simulink library "SimscapeCustomComponents_lib"  (R2025b)
settings: Solver=VariableStepAuto  StartTime=0.0  StopTime=10.0  RelTol=1e-3
undefined symbols (not defined in the file or in its folder): base, baseVdc, capacity, DiscIntNeverNeededParam, ee_sli_rtmsupport, filterInductance, freqeuncy, frequency, gcbh, gflInverter, gfmInverter, iMaxPU, Inertia, initialSOC, plantRating, solar, Ts, ups, Vac, windSystem, windTurbine
libraries: fl_lib x397, nesl_utility x171, eeGeneralControl x85, ee_lib x82, simulink x72, datacenter_lib x68, eeTransforms x38, slpidlib x24, buildingEnergy_lib x20, SimscapeFluids_lib x17, eeSinusoidalMeasurementV2 x8, eePwmGenerator x8
(part 23 of 24)

== system SimscapeCustomComponents_lib/Microgrid and Renewables/Sources/Solar Plant Integrated/Detailed/PV Plant & Controller/Controller/MPPT/Solar PV Controller/DC voltage controller & current reference/Current limits ==
  Imax : Inport
  idref : Inport  Port=2
  Sqrt1 : Sqrt
  Square3 : Math  Operator=square
  Square4 : Math  Operator=square
  Sum9 : Sum  Inputs=|+-
  iubd : Outport
  iubq : Outport  Port=2
  wires:
  Sum9/1 -> Sqrt1/1
  Square3/1 -> Sum9/1
  Square4/1 -> Sum9/2
  Imax/1 -> iubd/1, Square3/1
  Sqrt1/1 -> iubq/1
  idref/1 -> Square4/1

== system SimscapeCustomComponents_lib/Microgrid and Renewables/Sources/Solar Plant Integrated/Detailed/PV Plant & Controller/Controller/MPPT/Solar PV Controller/DC voltage controller & current reference/If Action Subsystem ==
  note: iq_ref_generator
  note: id_ref_generator
  Q ref : Inport
  Vmag : Inport  Port=2
  P pv : Inport  Port=3
  vdc : Inport  Port=4
  vdc ref : Inport  Port=5
  Action Port : ActionPort
  Subsystem : Subsystem
  Subsystem1 : Subsystem
  iq ref : Outport
  id ref : Outport  Port=2
  wires:
  [ubid] -> Subsystem1/5(id ub)
  [ubiq] -> Subsystem/2(iq ub)
  P pv/1 -> Subsystem1/2(P pv)
  Q ref/1 -> Subsystem/3(Q ref)
  vdc/1 -> Subsystem1/3(vdc)
  Vmag/1 -> Subsystem1/1(Vmag), Subsystem/1(V mag)
  vdc ref/1 -> Subsystem1/4(vdc ref)
  Subsystem1/1(idref) -> id ref/1
  Subsystem/1(iqref) -> iq ref/1

== system SimscapeCustomComponents_lib/Microgrid and Renewables/Sources/Solar Plant Integrated/Detailed/PV Plant & Controller/Controller/MPPT/Solar PV Controller/DC voltage controller & current reference/Subsystem ==
  V mag : Inport
  iq ub : Inport  Port=2
  Q ref : Inport  Port=3
  Constant : Constant  Value=1e-3
  Data Type Conversion Inherited : simulink/Signal Attributes/Data Type Conversion Inherited  ConvertRealWorld=Real World Value  DoSatur=off
  Divide2 : Product  Inputs=*/
  Gain1 : Gain  Gain=-1
  Gain3 : Gain  Gain=-1
  Saturation Dynamic2 : simulink/Discontinuities/Saturation Dynamic  OutMin=[]  OutMax=[]  OutDataTypeStr=Inherit: Same as second input  OutDataType=fixdt(1, 16)  OutScaling=2^-10  DoSatur=off
  Scope : Scope  NumInputPorts=3
      settings: ActiveDisplayYMinimum=1.32868  ActiveDisplayYMaximum=1.39248  DataLoggingVariableName=ScopeData8
  Switch : Switch  Criteria=u2 ~= 0  SaturateOnIntegerOverflow=off  InputSameDT=off
  iq ub1 : InportShadow  Port=2
  iqref : Outport
  wires:
  iq ub1/1 -> Gain3/1
  Divide2/1 -> Saturation Dynamic2/2, Scope/2
  Q ref/1 -> Divide2/1
  Gain3/1 -> Saturation Dynamic2/3, Scope/3
  iq ub/1 -> Saturation Dynamic2/1, Scope/1
  Saturation Dynamic2/1 -> Gain1/1
  V mag/1 -> Data Type Conversion Inherited/1, Switch/2, Switch/1
  Switch/1 -> Divide2/2
  Constant/1 -> Data Type Conversion Inherited/2
  Data Type Conversion Inherited/1 -> Switch/3
  Gain1/1 -> iqref/1

== system SimscapeCustomComponents_lib/Microgrid and Renewables/Sources/Solar Plant Integrated/Detailed/PV Plant & Controller/Controller/MPPT/Solar PV Controller/DC voltage controller & current reference/Subsystem1 ==
  Vmag : Inport
  P pv : Inport  Port=2
  vdc : Inport  Port=3
  vdc ref : Inport  Port=4
  id ub : Inport  Port=5
  Constant : Constant  Value=1e-3
  Constant4 : Constant  Value=0
  Data Type Conversion Inherited : simulink/Signal Attributes/Data Type Conversion Inherited  ConvertRealWorld=Real World Value  DoSatur=off
  Divide : Product  Inputs=/*
  Gain4 : Gain  Gain=1/(mVAbase)
  Saturation Dynamic1 : simulink/Discontinuities/Saturation Dynamic  OutMin=[]  OutMax=[]  OutDataTypeStr=Inherit: Same as second input  OutDataType=fixdt(1, 16)  OutScaling=2^-10  DoSatur=off
  Scope : Scope  NumInputPorts=2
      settings: ActiveDisplayYMinimum=715.83213  ActiveDisplayYMaximum=1444.49375
  Scope1 : Scope  NumInputPorts=3
      settings: ActiveDisplayYMinimum=0.2  ActiveDisplayYMaximum=2.2  DataLoggingVariableName=ScopeData7
  Sum : Sum  Inputs=|++
  Switch : Switch  Criteria=u2 ~= 0  SaturateOnIntegerOverflow=off  InputSameDT=off
  V_dc_Controller1 : Subsystem
  idref : Outport
  wires:
  Constant4/1 -> Saturation Dynamic1/3
  P pv/1 -> Gain4/1
  V_dc_Controller1/1(Out1) -> Sum/2
  Sum/1 -> Saturation Dynamic1/2, Scope1/2
  vdc ref/1 -> V_dc_Controller1/2(vdc ref), Scope/2
  id ub/1 -> Scope1/1, Saturation Dynamic1/1
  Gain4/1 -> Divide/2
  Divide/1 -> Sum/1
  Saturation Dynamic1/1 -> idref/1, Scope1/3
  vdc/1 -> V_dc_Controller1/1(vdc), Scope/1
  Vmag/1 -> Data Type Conversion Inherited/1, Switch/2, Switch/1
  Switch/1 -> Divide/1
  Constant/1 -> Data Type Conversion Inherited/2
  Data Type Conversion Inherited/1 -> Switch/3

== system SimscapeCustomComponents_lib/Microgrid and Renewables/Sources/Solar Plant Integrated/Detailed/PV Plant & Controller/Controller/MPPT/Solar PV Controller/PLL & Measurements/Subsystem ==
  abc : Inport
  Demux : Demux  Outputs=3
  Park Transform : eeTransforms/Park Transform  AxisAlignment=Q-axis  PowerInvariant=off
  "Sinusoidal Measurement (PLL, Three-Phase)" : eeSinusoidalMeasurementV2/Sinusoidal Measurement (PLL, Three-Phase)  InputFilter=on  InputNormalization=off  Kp_LF=Kppll  Ki_LF=Kipll  F0=frequency  Theta0=initialPhase  Ts=sampleTime
  Terminator : Terminator
  mag : Outport
  freq : Outport  Port=2
  angle : Outport  Port=3
  Vd : Outport  Port=4
  Vq : Outport  Port=5
  wires:
  "Sinusoidal Measurement (PLL, Three-Phase)"/2 -> angle/1, Park Transform/2
  Demux/3 -> Terminator/1
  abc/1 -> Park Transform/1, "Sinusoidal Measurement (PLL, Three-Phase)"/1
  Park Transform/1 -> Demux/1
  Demux/1 -> Vd/1
  Demux/2 -> Vq/1
  "Sinusoidal Measurement (PLL, Three-Phase)"/1 -> freq/1
  "Sinusoidal Measurement (PLL, Three-Phase)"/3 -> mag/1

== system SimscapeCustomComponents_lib/Microgrid and Renewables/Sources/Solar Plant Integrated/Detailed/PV Plant & Controller/Controller/MPPT/Solar PV Controller/Variant Subsystem/INC MPP ==
  Ipv : Inport
  Vpv : Inport  Port=2
  Abs : Abs  SaturateOnIntegerOverflow=off
  Add : Sum
  Constant : Constant  Value=0  SampleTime=sampleTime
  Constant1 : Constant  Value=delV  SampleTime=sampleTime
  Data Type Conversion Inherited : simulink/Signal Attributes/Data Type Conversion Inherited  ConvertRealWorld=Real World Value  DoSatur=off
  Data Type Conversion Inherited1 : simulink/Signal Attributes/Data Type Conversion Inherited  ConvertRealWorld=Real World Value  DoSatur=off
  Divide : Product  Inputs=*/
  Divide1 : Product  Inputs=*/
  Filtered Derivative (Discrete or Continuous) : eeGeneralControl/Filtered Derivative (Discrete or Continuous)  K=1  T=tSettling*2  B=inf  A=-inf  minRatio=1  init_option=Inherited from block input  x0=0  Ts=sampleTime
  Filtered Derivative (Discrete or Continuous)1 : eeGeneralControl/Filtered Derivative (Discrete or Continuous)  K=1  T=tSettling*2  B=inf  A=-inf  minRatio=1  init_option=Inherited from block input  x0=0  Ts=sampleTime
  Subtract5 : Sum  Inputs=-+
  Sum2 : Sum  Inputs=|++
  Switch : Switch  Criteria=u2 ~= 0  SaturateOnIntegerOverflow=off  InputSameDT=off
  Switch1 : Switch  Criteria=u2 > Threshold  SaturateOnIntegerOverflow=off  InputSameDT=off
  Switch4 : Switch  Criteria=u2 > Threshold  Threshold=1e-2  SaturateOnIntegerOverflow=off  InputSameDT=off
  Switch5 : Switch  Criteria=u2 > Threshold  SaturateOnIntegerOverflow=off  InputSameDT=off
  start MPPT Voltage : Constant  Value=Vdc  SampleTime=sampleTime
  Vmpp : Outport  VectorParamsAs1DForOutWhenUnconnected=off
  wires:
  Ipv/1 -> Filtered Derivative (Discrete or Continuous)/1, Divide1/1
  Switch5/1 -> Data Type Conversion Inherited1/1, Add/1, Subtract5/2
  Vpv/1 -> Filtered Derivative (Discrete or Continuous)1/1, Divide1/2, Data Type Conversion Inherited/1, Switch5/2, Switch5/1
  Add/1 -> [Vinc]  "INC"
  Subtract5/1 -> [Vdec]  "DEC"
  Filtered Derivative (Discrete or Continuous)/1 -> Switch/3, Divide/1
  Divide/1 -> Sum2/1
  Divide1/1 -> Sum2/2
  Sum2/1 -> Switch/1
  Switch/1 -> Switch1/2, Abs/1
  [Vinc] -> Switch1/1
  [Vdec] -> Switch1/3
  Filtered Derivative (Discrete or Continuous)1/1 -> Switch/2, Divide/2
  Abs/1 -> Switch4/2
  Constant/1 -> Switch4/3
  Constant1/1 -> Switch4/1
  Switch1/1 -> Vmpp/1
  Data Type Conversion Inherited/1 -> Switch5/3
  start MPPT Voltage/1 -> Data Type Conversion Inherited/2
  Switch4/1 -> Data Type Conversion Inherited1/2
  Data Type Conversion Inherited1/1 -> Add/2, Subtract5/1

== system SimscapeCustomComponents_lib/Microgrid and Renewables/Sources/Solar Plant Integrated/Detailed/PV Plant & Controller/Controller/MPPT/Solar PV Controller/Variant Subsystem/P&O MPP ==
  Ipv : Inport
  Vpv : Inport  Port=2
  AND1 : Logic  IconShape=distinctive  AllPortsSameDT=off  OutDataTypeStr=boolean
  Add : Sum
  Compare To Zero1 : simulink/Logic and Bit Operations/Compare To Zero  relop=>=  OutDataTypeStr=boolean
  Compare To Zero2 : simulink/Logic and Bit Operations/Compare To Zero  relop=>=  OutDataTypeStr=boolean
  Constant1 : Constant  Value=delV  SampleTime=sampleTime
  Data Type Conversion Inherited : simulink/Signal Attributes/Data Type Conversion Inherited  ConvertRealWorld=Real World Value  DoSatur=off
  Data Type Conversion Inherited1 : simulink/Signal Attributes/Data Type Conversion Inherited  ConvertRealWorld=Real World Value  DoSatur=off
  Filtered Derivative (Discrete or Continuous) : eeGeneralControl/Filtered Derivative (Discrete or Continuous)  K=1  T=tSettling*2  B=inf  A=-inf  minRatio=1  init_option=Inherited from block input  x0=0  Ts=sampleTime
  Filtered Derivative (Discrete or Continuous)1 : eeGeneralControl/Filtered Derivative (Discrete or Continuous)  K=1  T=tSettling*2  B=inf  A=-inf  minRatio=1  init_option=Inherited from block input  x0=0  Ts=sampleTime
  NOR : Logic  Operator=NOR  IconShape=distinctive  AllPortsSameDT=off  OutDataTypeStr=boolean
  OR : Logic  Operator=OR  IconShape=distinctive  AllPortsSameDT=off  OutDataTypeStr=boolean
  Product : Product
  Subtract5 : Sum  Inputs=-+
  Switch4 : Switch  Criteria=u2 ~= 0  SaturateOnIntegerOverflow=off  InputSameDT=off
  Switch5 : Switch  Criteria=u2 > Threshold  SaturateOnIntegerOverflow=off  InputSameDT=off
  start MPPT Voltage : Constant  Value=Vdc  SampleTime=sampleTime
  Vmpp : Outport  VectorParamsAs1DForOutWhenUnconnected=off
  wires:
  OR/1 -> Switch4/2
  Compare To Zero1/1 -> NOR/1, AND1/2
  Compare To Zero2/1 -> NOR/2, AND1/1
  Switch5/1 -> Data Type Conversion Inherited1/1, Add/1, Subtract5/2
  Constant1/1 -> Data Type Conversion Inherited1/2
  Vpv/1 -> Product/2, Filtered Derivative (Discrete or Continuous)1/1, Data Type Conversion Inherited/1, Switch5/2, Switch5/1
  Add/1 -> [Vinc]  "INC"
  NOR/1 -> OR/2
  Subtract5/1 -> [Vdec]  "DEC"
  [Vdec] -> Switch4/3
  Filtered Derivative (Discrete or Continuous)1/1 -> Compare To Zero1/1
  Filtered Derivative (Discrete or Continuous)/1 -> Compare To Zero2/1
  AND1/1 -> OR/1
  [Vinc] -> Switch4/1
  Ipv/1 -> Product/1
  Product/1 -> Filtered Derivative (Discrete or Continuous)/1
  Switch4/1 -> Vmpp/1
  Data Type Conversion Inherited/1 -> Switch5/3
  start MPPT Voltage/1 -> Data Type Conversion Inherited/2
  Data Type Conversion Inherited1/1 -> Add/2, Subtract5/1

== system SimscapeCustomComponents_lib/Microgrid and Renewables/Sources/Solar Plant Integrated/Detailed/PV Plant & Controller/Controller/Power Reference/Power Reference Controller/PLL & Measurements/Measurement1 ==
  u : Inport
  Lead-Lag (Discrete or Continuous) : eeGeneralControl/Lead-Lag (Discrete or Continuous)  T1=0  T2=1e-3  B=inf  A=-inf  init_option=Inherited from block input  x0=0  Ts=Ts
  Vg : Outport
  wires:
  Lead-Lag (Discrete or Continuous)/1 -> Vg/1
  u/1 -> Lead-Lag (Discrete or Continuous)/1

== system SimscapeCustomComponents_lib/Microgrid and Renewables/Sources/Solar Plant Integrated/Detailed/PV Plant & Controller/Controller/Power Reference/Power Reference Controller/PLL & Measurements/Measurement2 ==
  u : Inport
  Lead-Lag (Discrete or Continuous) : eeGeneralControl/Lead-Lag (Discrete or Continuous)  T1=0  T2=1e-3  B=inf  A=-inf  init_option=Inherited from block input  x0=0  Ts=Ts
  Vg : Outport
  wires:
  Lead-Lag (Discrete or Continuous)/1 -> Vg/1
  u/1 -> Lead-Lag (Discrete or Continuous)/1

== system SimscapeCustomComponents_lib/Microgrid and Renewables/Sources/Solar Plant Integrated/Detailed/PV Plant & Controller/Controller/Power Reference/Power Reference Controller/PLL & Measurements/Subsystem ==
  Vabc : Inport
  Iabc : Inport  Port=2
  Demux : Demux  Outputs=3
  Demux1 : Demux  Outputs=3
  Park Transform : eeTransforms/Park Transform  AxisAlignment=Q-axis  PowerInvariant=off
  Park Transform1 : eeTransforms/Park Transform  AxisAlignment=Q-axis  PowerInvariant=off
  Scope : Scope  NumInputPorts=2
      settings: ActiveDisplayYMinimum=0.97158  ActiveDisplayYMaximum=1.00612  DataLoggingVariableName=ScopeData5
  "Sinusoidal Measurement (PLL, Three-Phase)" : eeSinusoidalMeasurementV2/Sinusoidal Measurement (PLL, Three-Phase)  InputFilter=on  InputNormalization=off  Kp_LF=kpPLL  Ki_LF=kiPLL  F0=frequency  Theta0=0  Ts=-1
  Terminator : Terminator
  Terminator1 : Terminator
  mag : Outport
  freq : Outport  Port=2
  angle : Outport  Port=3
  Vd : Outport  Port=4
  Vq : Outport  Port=5
  Id1 : Outport  Port=6
  Iq1 : Outport  Port=7
  wires:
  Demux/3 -> Terminator/1
  Vabc/1 -> Park Transform/1, "Sinusoidal Measurement (PLL, Three-Phase)"/1
  Park Transform/1 -> Demux/1
  Demux/1 -> Scope/1, Vd/1
  Demux/2 -> Scope/2, Vq/1
  "Sinusoidal Measurement (PLL, Three-Phase)"/2 -> angle/1, Park Transform1/2, Park Transform/2
  "Sinusoidal Measurement (PLL, Three-Phase)"/1 -> freq/1
  "Sinusoidal Measurement (PLL, Three-Phase)"/3 -> mag/1
  Park Transform1/1 -> Demux1/1
  Demux1/1 -> Id1/1
  Demux1/2 -> Iq1/1
  Demux1/3 -> Terminator1/1
  Iabc/1 -> Park Transform1/1

== system SimscapeCustomComponents_lib/Microgrid and Renewables/Sources/Solar Plant Integrated/Detailed/PV Plant & Controller/Controller/Power Reference/Power Reference Controller/Power Reference Controller/Current_controller ==
  id-ref : Inport
  ipvd : Inport  Port=2
  iqref : Inport  Port=3
  iq : Inport  Port=4
  Vd : Inport  Port=5
  Vq : Inport  Port=6
  Constant4 : Constant  Value=0
  Gain1 : Gain  Gain=2*1*pi*60*L/zbase
  Gain2 : Gain  Gain=2*1*pi*60*L/zbase
  Mux1 : Mux  Inputs=3
  PID Controller : slpidlib/PID Controller  Controller=PID  Form=Parallel  TimeDomain=Discrete-time  UseExternalTs=off  SampleTime=-1  IntegratorMethod=Forward Euler  FilterMethod=Forward Euler  ControllerParametersSource=internal  P=Kpic  I=Kiic  UseKiTs=off  D=Kd  UseExternalDerivativeSource=off  N=100  UseFilter=on  TunerSelectOption=Transfer Function Based (PID Tuner App)  InitialConditionSource=internal  InitialConditionForIntegrator=0  InitialConditionForFilter=0  DifferentiatorICPrevScaledInput=0  ExternalReset=none  TrackingMode=off  Kt=1  LimitOutput=on  SatLimitsSource=internal  UpperSaturationLimit=3  LowerSaturationLimit=-3  LinearizeAsGain=on  AntiWindupMode=clamping  Kb=1  LimitIntegrator=on  UpperIntegratorSaturationLimit=3  LowerIntegratorSaturationLimit=-3  POutMin=[]  POutMax=[]  IOutMin=[]  IOutMax=[]  DOutMin=[]  DOutMax=[]  NOutMin=[]  NOutMax=[]  SumOutMin=[]  SumOutMax=[]  SaturationOutMin=[]  SaturationOutMax=[]  PParamMin=[]  PParamMax=[]  IParamMin=[]  IParamMax=[]  DParamMin=[]  DParamMax=[]  NParamMin=[]  NParamMax=[]  KbParamMin=[]  KbParamMax=[]  KtParamMin=[]  KtParamMax=[]  KbOutMin=[]  KbOutMax=[]  KtOutMin=[]  KtOutMax=[]  IntegratorOutMin=[]  IntegratorOutMax=[]  FilterOutMin=[]  FilterOutMax=[]  SumI1OutMin=[]  SumI1OutMax=[]  SumI2OutMin=[]  SumI2OutMax=[]  SumI3OutMin=[]  SumI3OutMax=[]  SumI4OutMin=[]  SumI4OutMax=[]  SumDOutMin=[]  SumDOutMax=[]  DifferentiatorOutMin=[]  DifferentiatorOutMax=[]  FilterDiffOutCoefMin=[]  FilterDiffOutCoefMax=[]  ReciprocalOutMin=[]  ReciprocalOutMax=[]  SumDenOutMin=[]  SumDenOutMax=[]  SumNumOutMin=[]  SumNumOutMax=[]  DivideOutMin=[]  DivideOutMax=[]  UdiffTsProdOutMin=[]  UdiffTsProdOutMax=[]  NTsProdOutMin=[]  NTsProdOutMax=[]  UintegralTsProdOutMin=[]  UintegralTsProdOutMax=[]  UngainTsProdOutMin=[]  UngainTsProdOutMax=[]  ClampingZeroOutDataTypeStr=Inherit: Inherit via back propagation  ClampingZeroOutMin=[]  ClampingZeroOutMax=[]  FilterDenConstantOutDataTypeStr=Inherit: Inherit via back propagation  FilterDenConstantOutMin=[]  FilterDenConstantOutMax=[]  PCopyOutDataTypeStr=Inherit: Inherit via back propagation  PCopyOutMin=[]  PCopyOutMax=[]  NCopyOutDataTypeStr=Inherit: Inherit via back propagation  NCopyOutMin=[]  NCopyOutMax=[]  IntegratorContinuousStateAttributes=''  IntegratorStateMustResolveToSignalObject=off  IntegratorRTWStateStorageClass=Auto  FilterContinuousStateAttributes=''  FilterStateMustResolveToSignalObject=off  FilterRTWStateStorageClass=Auto  ParallelPVariant=InternalParameters  IdealPVariant=Disabled  IVariant=InternalParameters  DVariant=InternalParameters  IntegratorVariant=Discrete  SatVariant=Enabled  AWVariant=DiscClampingParallel  PCopyVariant=Disabled  TRVariant=Disabled  FdbkBlocksVariant=Forward  IdealPFdbkVariant=Disabled  SatFdbkVariant=Disabled  DerivativeFilterVariant=ForwardEulerFilter  NVariant=InternalParameters  NCopyVariant=Disabled  FilterICVariant=InternalICsFilter  IntegratorICVariant=InternalICs  ExternalResetVariant=Disabled  TRSumVariant=Passthrough  SumFdbkVariant=Disabled  SumVariant=Sum_PID  TsampFilterVariant=InternalTs  TsampNgainVariant=Passthrough  TsampIntegralVariant=Disabled_SignalSpec  ExternalSaturationOutDataTypeStr=Inherit: Same as second input  DerivativeSourceVariant=ErrorSignal  PreIntVariant=InternalPreInt
  PID Controller1 : slpidlib/PID Controller  Controller=PID  Form=Parallel  TimeDomain=Discrete-time  UseExternalTs=off  SampleTime=-1  IntegratorMethod=Forward Euler  FilterMethod=Forward Euler  ControllerParametersSource=internal  P=Kpic  I=Kiic  UseKiTs=off  D=Kd  UseExternalDerivativeSource=off  N=100  UseFilter=on  TunerSelectOption=Transfer Function Based (PID Tuner App)  InitialConditionSource=internal  InitialConditionForIntegrator=0  InitialConditionForFilter=0  DifferentiatorICPrevScaledInput=0  ExternalReset=none  TrackingMode=off  Kt=1  LimitOutput=on  SatLimitsSource=internal  UpperSaturationLimit=3  LowerSaturationLimit=-3  LinearizeAsGain=on  AntiWindupMode=clamping  Kb=1  LimitIntegrator=on  UpperIntegratorSaturationLimit=3  LowerIntegratorSaturationLimit=-3  POutMin=[]  POutMax=[]  IOutMin=[]  IOutMax=[]  DOutMin=[]  DOutMax=[]  NOutMin=[]  NOutMax=[]  SumOutMin=[]  SumOutMax=[]  SaturationOutMin=[]  SaturationOutMax=[]  PParamMin=[]  PParamMax=[]  IParamMin=[]  IParamMax=[]  DParamMin=[]  DParamMax=[]  NParamMin=[]  NParamMax=[]  KbParamMin=[]  KbParamMax=[]  KtParamMin=[]  KtParamMax=[]  KbOutMin=[]  KbOutMax=[]  KtOutMin=[]  KtOutMax=[]  IntegratorOutMin=[]  IntegratorOutMax=[]  FilterOutMin=[]  FilterOutMax=[]  SumI1OutMin=[]  SumI1OutMax=[]  SumI2OutMin=[]  SumI2OutMax=[]  SumI3OutMin=[]  SumI3OutMax=[]  SumI4OutMin=[]  SumI4OutMax=[]  SumDOutMin=[]  SumDOutMax=[]  DifferentiatorOutMin=[]  DifferentiatorOutMax=[]  FilterDiffOutCoefMin=[]  FilterDiffOutCoefMax=[]  ReciprocalOutMin=[]  ReciprocalOutMax=[]  SumDenOutMin=[]  SumDenOutMax=[]  SumNumOutMin=[]  SumNumOutMax=[]  DivideOutMin=[]  DivideOutMax=[]  UdiffTsProdOutMin=[]  UdiffTsProdOutMax=[]  NTsProdOutMin=[]  NTsProdOutMax=[]  UintegralTsProdOutMin=[]  UintegralTsProdOutMax=[]  UngainTsProdOutMin=[]  UngainTsProdOutMax=[]  ClampingZeroOutDataTypeStr=Inherit: Inherit via back propagation  ClampingZeroOutMin=[]  ClampingZeroOutMax=[]  FilterDenConstantOutDataTypeStr=Inherit: Inherit via back propagation  FilterDenConstantOutMin=[]  FilterDenConstantOutMax=[]  PCopyOutDataTypeStr=Inherit: Inherit via back propagation  PCopyOutMin=[]  PCopyOutMax=[]  NCopyOutDataTypeStr=Inherit: Inherit via back propagation  NCopyOutMin=[]  NCopyOutMax=[]  IntegratorContinuousStateAttributes=''  IntegratorStateMustResolveToSignalObject=off  IntegratorRTWStateStorageClass=Auto  FilterContinuousStateAttributes=''  FilterStateMustResolveToSignalObject=off  FilterRTWStateStorageClass=Auto  ParallelPVariant=InternalParameters  IdealPVariant=Disabled  IVariant=InternalParameters  DVariant=InternalParameters  IntegratorVariant=Discrete  SatVariant=Enabled  AWVariant=DiscClampingParallel  PCopyVariant=Disabled  TRVariant=Disabled  FdbkBlocksVariant=Forward  IdealPFdbkVariant=Disabled  SatFdbkVariant=Disabled  DerivativeFilterVariant=ForwardEulerFilter  NVariant=InternalParameters  NCopyVariant=Disabled  FilterICVariant=InternalICsFilter  IntegratorICVariant=InternalICs  ExternalResetVariant=Disabled  TRSumVariant=Passthrough  SumFdbkVariant=Disabled  SumVariant=Sum_PID  TsampFilterVariant=InternalTs  TsampNgainVariant=Passthrough  TsampIntegralVariant=Disabled_SignalSpec  ExternalSaturationOutDataTypeStr=Inherit: Same as second input  DerivativeSourceVariant=ErrorSignal  PreIntVariant=InternalPreInt
  Saturation : Saturate  UpperLimit=1.2  LowerLimit=-1.2
  Saturation1 : Saturate  UpperLimit=1.2  LowerLimit=-1.2
  Scope : Scope  NumInputPorts=2
      settings: ActiveDisplayYMinimum=0.49995  ActiveDisplayYMaximum=0.50039
  Scope1 : Scope  NumInputPorts=2
      settings: ActiveDisplayYMinimum=-1  ActiveDisplayYMaximum=1  DataLoggingVariableName=ScopeData2
  Scope2 : Scope  NumInputPorts=3
      settings: ActiveDisplayYMinimum=0.92426  ActiveDisplayYMaximum=1.0261  DataLoggingVariableName=ScopeData2
  Sum1 : Sum  Inputs=|+-
  Sum3 : Sum  Inputs=|++-
  Sum4 : Sum  Inputs=|+++
  Sum5 : Sum  Inputs=|+-
  mdq0 : Outport
  wires:
  PID Controller/1 -> Scope2/2, Sum3/2
  Sum3/1 -> Saturation/1, [Ed]
  Gain2/1 -> Scope2/3, Sum3/3
  ipvd/1 -> Scope/2, Gain1/1, Sum1/2
  id-ref/1 -> Scope/1, Sum1/1
  Gain1/1 -> Sum4/3
  Vq/1 -> Sum4/2
  iq/1 -> Scope1/2, Gain2/1, Sum5/2
  Sum1/1 -> PID Controller/1
  Constant4/1 -> Mux1/3
  Sum5/1 -> PID Controller1/1
  PID Controller1/1 -> Sum4/1
  Sum4/1 -> Saturation1/1, [Eq]
  Mux1/1 -> mdq0/1
  iqref/1 -> Scope1/1, Sum5/1
  Saturation/1 -> Mux1/1
  Saturation1/1 -> Mux1/2
  Vd/1 -> Scope2/1, Sum3/1

== system SimscapeCustomComponents_lib/Microgrid and Renewables/Sources/Solar Plant Integrated/Detailed/PV Plant & Controller/Controller/Power Reference/Power Reference Controller/Power Reference Controller/Reference Current ==
  note: Current Limiters
  note: Avoid division by zero during start
  V-mag : Inport
  LVRT_iq : Inport  Port=2
  PRef : Inport  Port=3
  QRef : Inport  Port=4
  Constant1 : Constant
  Constant3 : Constant  Value=Imax
  Current limits : Subsystem
  Refernce id generation : Subsystem
  Refernce iq generation : Subsystem
  Switch : Switch  Criteria=u2 ~= 0  SaturateOnIntegerOverflow=off  InputSameDT=off
  Unit Delay1 : UnitDelay  SampleTime=Ts
  Unit Delay3 : UnitDelay  SampleTime=Ts
  id_ref : Outport
  iq_ref : Outport  Port=2
  wires:
  Unit Delay1/1 -> Current limits/2(iqref)
  Current limits/1(iubq) -> Refernce iq generation/1(ubiq)
  Unit Delay3/1 -> Current limits/3(idref)
  Constant3/1 -> Current limits/1(Imax)
  Refernce id generation/1(id_ref) -> id_ref/1, Unit Delay3/1
  Refernce iq generation/1(iq_ref) -> Unit Delay1/1, iq_ref/1
  LVRT_iq/1 -> Refernce iq generation/3(LVRT_iq)
  V-mag/1 -> Switch/1, Switch/2
  Switch/1 -> Refernce id generation/1(V_mag), Refernce iq generation/2(V_mag)
  Constant1/1 -> Switch/3
  QRef/1 -> Refernce iq generation/4(Q_ref)
  PRef/1 -> Refernce id generation/3(PRef)
  Current limits/2(iubd) -> Refernce id generation/2(ubid)

== system SimscapeCustomComponents_lib/Microgrid and Renewables/Sources/Wind Plant Integrated/Detailed/Wind Turbine and Converters/Wind Controller/Wind Grid-side Converter Controller/DC voltage controller & current reference/Subsystem1/V_dc_Controller1 ==
  Wind_plant1 : Inport
  In2 : Inport  Port=2
  Gain : Gain  Gain=1/Vdc
  PI : Subsystem
  Sum : Sum  Inputs=|+-
  Out1 : Outport
  wires:
  Wind_plant1/1 -> Sum/1
  In2/1 -> Sum/2
  Sum/1 -> Gain/1
  Gain/1 -> PI/1(Input)
  PI/1(Out2) -> Out1/1

== system SimscapeCustomComponents_lib/Microgrid and Renewables/Sources/Wind Plant Integrated/Detailed/Wind Turbine and Converters/Wind Plant/Back-to-Back Converters/Switching/Grid Side Converter/Pulse Generation1 ==
  G : Inport
  Constant : Constant  Value=5
  Subtract : Sum  Inputs=-+
  G1 : Outport  VectorParamsAs1DForOutWhenUnconnected=off
  G2 : Outport  Port=2  VectorParamsAs1DForOutWhenUnconnected=off
  wires:
  Subtract/1 -> G2/1
  Constant/1 -> Subtract/2
  G/1 -> G1/1, Subtract/1

== system SimscapeCustomComponents_lib/Microgrid and Renewables/Sources/Wind Plant Integrated/Detailed/Wind Turbine and Converters/Wind Plant/Back-to-Back Converters/Switching/Machine Side Converter/Pulse Generation ==
  G : Inport
  Constant : Constant  Value=5
  Subtract : Sum  Inputs=-+
  G1 : Outport  VectorParamsAs1DForOutWhenUnconnected=off
  G2 : Outport  Port=2  VectorParamsAs1DForOutWhenUnconnected=off
  wires:
  Subtract/1 -> G2/1
  Constant/1 -> Subtract/2
  G/1 -> G1/1, Subtract/1

== system SimscapeCustomComponents_lib/Microgrid and Renewables/Storage/BESS Integrated/Detailed/BESS Controller/Grid Forming/Current Limiting/CurrentLimitingMethod/currentLimitAndVirtual/Current Saturation ==
  note: Vs-delV
  Id : Inport
  Iq : Inport  Port=2
  Imaxsat : Inport  Port=3
  Enable : EnablePort
  Compare : Subsystem
  Constant1 : Constant  Value=0
  Constant2 : Constant  Value=0
  If : If
  If Action Subsystem : Subsystem  TreatAsAtomicUnit=on
  If Action Subsystem1 : Subsystem  TreatAsAtomicUnit=on
  Math Function : Math  Operator=hypot
  Merge : Merge
  Merge1 : Merge
  Subtract : Sum  Inputs=+-
  delVd : Outport
  delVq : Outport  Port=2
  idmax : Outport  Port=3
  iqmax : Outport  Port=4
  wires:
  Iq/1 -> [Isq], Math Function/2
  If/1 -> If Action Subsystem/Action
  If Action Subsystem1/1(Idmax) -> Merge/2
  Constant2/1 -> delVq/1
  Math Function/1 -> [Is], Subtract/2
  If/2 -> If Action Subsystem1/Action
  If Action Subsystem/2(Iqmax) -> Merge1/1
  Subtract/1 -> Compare/1(u)
  Compare/1(Out1) -> If/1
  If Action Subsystem/1(Idmax) -> Merge/1
  [Is] -> If Action Subsystem/1(Is)
  Id/1 -> [Isd], Math Function/1
  If Action Subsystem1/2(Iqmax) -> Merge1/2
  Merge/1 -> idmax/1
  [Isd] -> If Action Subsystem/2(Isd)
  Constant1/1 -> delVd/1
  [Isq] -> If Action Subsystem/3(Isq)
  Merge1/1 -> iqmax/1
  Imaxsat/1 -> [Imax], Subtract/1
  [Imax] -> If Action Subsystem/4(maxI)

== system SimscapeCustomComponents_lib/Microgrid and Renewables/Storage/BESS Integrated/Detailed/BESS Controller/Grid Forming/Current Limiting/CurrentLimitingMethod/currentLimitAndVirtual/No Fault Ride Through ==
  Id : Inport
  Iq : Inport  Port=2
  Enable : EnablePort
  Constant{1..4} (4 alike) : Constant  Value=0
  Terminator : Terminator
  Terminator1 : Terminator
  delVd : Outport
  delVq : Outport  Port=2
  idmax : Outport  Port=3
  iqmax : Outport  Port=4
  wires:
  Constant3/1 -> iqmax/1
  Constant2/1 -> idmax/1
  Constant1/1 -> delVd/1
  Constant4/1 -> delVq/1
  Id/1 -> Terminator/1
  Iq/1 -> Terminator1/1

== system SimscapeCustomComponents_lib/Microgrid and Renewables/Storage/BESS Integrated/Detailed/BESS Controller/Grid Forming/Current Limiting/CurrentLimitingMethod/currentLimitAndVirtual/VI ==
  note: Resistance coefficient
  note: X/R ratio
  Id : Inport
  Iq : Inport  Port=2
  Imax : Inport  Port=3
  Enable : EnablePort
  Constant1 : Constant  Value=0
  Constant2 : Constant  Value=0
  Constant3 : Constant  Value=0
  Gain : Gain  Gain=ctLimitVirtualImp
  Gain1 : Gain  Gain=ctLimitXbyR
  Low-Pass Filter : eeGeneralControl/Low-Pass Filter (Discrete or Continuous)  K=1  T=currentVITimeConst  B=inf  A=-inf  init_option=Inherited from block input  x0=0  Ts=-1
  Math Function : Math  Operator=hypot
  Product{,1..3} (4 alike) : Product
  Relay1 : Relay  OnSwitchValue=0.01  OffSwitchValue=-0.1
  Saturation : Saturate  UpperLimit=1  LowerLimit=-1
  Saturation1 : Saturate  UpperLimit=1  LowerLimit=-1
  Sum : Sum  Inputs=|+-
  Sum1 : Sum  Inputs=|+-
  Sum2 : Sum  Inputs=++|
  Switch : Switch  Criteria=u2 > Threshold  SaturateOnIntegerOverflow=off  InputSameDT=off
  delVd : Outport
  delVq : Outport  Port=2
  idmax : Outport  Port=3
  iqmax : Outport  Port=4
  wires:
  Gain1/1 -> Product1/2, Product2/1
  Product3/1 -> Sum2/2
  Id/1 -> Math Function/1, [Igd]
  Sum2/1 -> Saturation1/1
  Sum/1 -> Gain/1, Relay1/1
  Sum1/1 -> Saturation/1
  Product/1 -> Sum1/1
  [Igq] -> Product3/1, Product2/2
  Iq/1 -> [Igq], Math Function/2
  Math Function/1 -> Low-Pass Filter/1  "Is"
  Switch/1 -> Product3/2, Product/1, Gain1/1
  [Igd] -> Product1/1, Product/2
  Saturation1/1 -> delVq/1
  Product1/1 -> Sum2/1
  Product2/1 -> Sum1/2
  Gain/1 -> Switch/1
  Constant1/1 -> Switch/3
  Saturation/1 -> delVd/1
  Constant3/1 -> iqmax/1
  Constant2/1 -> idmax/1
  Relay1/1 -> Switch/2
  Low-Pass Filter/1 -> Sum/1
  Imax/1 -> Sum/2  "IsMaximum"

== system SimscapeCustomComponents_lib/Microgrid and Renewables/Storage/BESS Integrated/Detailed/BESS Controller/Grid Forming/Current Limiting/CurrentLimitingMethod/currentSaturation/Compare ==
  u : Inport
  AND : Logic  IconShape=distinctive  AllPortsSameDT=off  OutDataTypeStr=boolean
  Compare To Constant : simulink/Logic and Bit Operations/Compare To Constant  relop=>  const=ctLimitDelayTime  OutDataTypeStr=boolean
  Compare To Zero : simulink/Logic and Bit Operations/Compare To Zero  relop=<=  OutDataTypeStr=boolean
  Data Type Conversion : DataTypeConversion  SaturateOnIntegerOverflow=off  RndMeth=Floor
  Data Type Conversion1 : DataTypeConversion  SaturateOnIntegerOverflow=off  RndMeth=Floor
  Discrete-Time Integrator : DiscreteIntegrator  IntegratorMethod=Integration: Backward Euler  ExternalReset=level  SampleTime=currentControlTs  LimitOutput=on  UpperSaturationLimit=ctLimitDelayTime*2  LowerSaturationLimit=0  ICPrevOutput=DiscIntNeverNeededParam  ICPrevScaledInput=DiscIntNeverNeededParam
  Out1 : Outport
  wires:
  AND/1 -> Data Type Conversion/1
  Compare To Zero/1 -> Data Type Conversion1/1
  Compare To Constant/1 -> AND/2
  u/1 -> Compare To Zero/1
  Discrete-Time Integrator/1 -> Compare To Constant/1
  Data Type Conversion/1 -> Out1/1
  Data Type Conversion1/1 -> Discrete-Time Integrator/2, Discrete-Time Integrator/1, AND/1

== system SimscapeCustomComponents_lib/Microgrid and Renewables/Storage/BESS Integrated/Detailed/BESS Controller/Grid Forming/Current Limiting/CurrentLimitingMethod/currentSaturation/If Action Subsystem ==
  Is : Inport
  Isd : Inport  Port=2
  Isq : Inport  Port=3
  Action Port : ActionPort
  Constant : Constant  Value=maxSatCurrentLimit
  Divide : Product  Inputs=*/
  Product : Product
  Product1 : Product
  Idmax : Outport
  Iqmax : Outport  Port=2
  wires:
  Constant/1 -> Divide/1
  Is/1 -> Divide/2
  Divide/1 -> Product1/2, Product/1
  Isd/1 -> Product1/1
  Isq/1 -> Product/2
  Product1/1 -> Idmax/1
  Product/1 -> Iqmax/1

== system SimscapeCustomComponents_lib/Microgrid and Renewables/Storage/BESS Integrated/Detailed/BESS Controller/Grid Forming/Current Limiting/CurrentLimitingMethod/currentSaturation/If Action Subsystem1 ==
  Action Port : ActionPort
  Constant3 : Constant  Value=0
  Constant4 : Constant  Value=0
  Idmax : Outport
  Iqmax : Outport  Port=2
  wires:
  Constant4/1 -> Iqmax/1
  Constant3/1 -> Idmax/1

== system SimscapeCustomComponents_lib/Microgrid and Renewables/Storage/BESS Integrated/Detailed/BESS Controller/Grid Forming/Grid Voltage Reactive Power Support/Modifying Reactive Power Reference/Changing the Power Reference/ActivePowerReference ==
  note: Ensure Pref sign is maintained
  Id : Inport
  Vd : Inport  Port=2
  Pref : Inport  Port=3
  Abs1 : Abs  SaturateOnIntegerOverflow=off
  Abs2 : Abs  SaturateOnIntegerOverflow=off
  Min : MinMax  Inputs=2
  Product : Product
  Product2 : Product
  Saturation : Saturate  UpperLimit=1  LowerLimit=-1
  Sign : Signum
  PrefNew : Outport
  wires:
  Pref/1 -> Abs1/1, Sign/1
  Id/1 -> Product/1
  Sign/1 -> Product2/2
  Abs1/1 -> Min/2
  Product/1 -> Abs2/1
  Min/1 -> Product2/1
  Product2/1 -> Saturation/1
  Abs2/1 -> Min/1
  Vd/1 -> Product/2
  Saturation/1 -> PrefNew/1

== system SimscapeCustomComponents_lib/Microgrid and Renewables/Storage/BESS Integrated/Detailed/BESS Controller/Grid Forming/Grid Voltage Reactive Power Support/Modifying Reactive Power Reference/Changing the Power Reference/EstimateIdForGivenIq ==
  Iq : Inport
  Add Constant1 : Bias  Bias=1*1  SaturateOnIntegerOverflow=off
  Gain : Gain  Gain=-1
  Gain3 : Gain  Gain=0.9
  Sqrt : Sqrt
  Square : Math  Operator=square
  Id : Outport
  wires:
  Square/1 -> Gain/1
  Gain3/1 -> Id/1
  Gain/1 -> Add Constant1/1
  Sqrt/1 -> Gain3/1
  Add Constant1/1 -> Sqrt/1
  Iq/1 -> Square/1

== system SimscapeCustomComponents_lib/Microgrid and Renewables/Storage/BESS Integrated/Detailed/BESS Controller/Grid Forming/Grid Voltage Reactive Power Support/Modifying Reactive Power Reference/Changing the Power Reference/EstimateIqForReactivePower ==
  note: Computing minimum reactive power as per GC0137
  Vmin : Inport
  Vd : Inport  Port=2
  Vs : Inport  Port=3
  Abs : Abs  SaturateOnIntegerOverflow=off
  Add : Sum
  Add Constant : Bias  Bias=1  SaturateOnIntegerOverflow=off
  GC0137 line slope : Gain  Gain=-1.4578
  Gain4 : Gain  Gain=1.5
  Saturation : Saturate  UpperLimit=1  LowerLimit=0
  Saturation1 : Saturate  UpperLimit=1  LowerLimit=-1
  Subtract : Sum  Inputs=+-
  Iq : Outport
  wires:
  Abs/1 -> GC0137 line slope/1
  GC0137 line slope/1 -> Add Constant/1
  Subtract/1 -> Gain4/1
  Saturation1/1 -> Add/1
  Gain4/1 -> Saturation1/1
  Vmin/1 -> Subtract/1
  Vs/1 -> Abs/1
  Vd/1 -> Subtract/2
  Add/1 -> Saturation/1
  Saturation/1 -> Iq/1
  Add Constant/1 -> Add/2

== system SimscapeCustomComponents_lib/Microgrid and Renewables/Storage/BESS Integrated/Detailed/BESS Controller/Grid Forming/Grid Voltage Reactive Power Support/Modifying Reactive Power Reference/Changing the Power Reference/ReactivePowerReference ==
  Vd : Inport
  Iq : Inport  Port=2
  Compute Power : Product
  Constant : Constant  Value=0.3
  Gain2 : Gain  Gain=1.05
  Switch : Switch  Criteria=u2 > Threshold  Threshold=0.3  SaturateOnIntegerOverflow=off  InputSameDT=off
  QrefNew : Outport
  wires:
  Compute Power/1 -> QrefNew/1
  Gain2/1 -> Compute Power/2
  Constant/1 -> Switch/3
  Iq/1 -> Gain2/1
  Vd/1 -> Switch/2, Switch/1
  Switch/1 -> Compute Power/1

== system SimscapeCustomComponents_lib/Microgrid and Renewables/Storage/BESS Integrated/Detailed/BESS Controller/Grid Forming/Measurement/Frequency Measurement/Frequency Measurement/If Action Subsystem ==
  V : Inport
  Time : Inport  Port=2
  Action Port : ActionPort
  Constant1 : Constant  Value=initialFrequency
  Delay : Delay  DelayLength=1
  Delay1 : Delay  DelayLength=1
  Frequency estimation : Subsystem  TreatAsAtomicUnit=on
  Hit Crossing : HitCross
  Second-Order Filter : eeGeneralControl/Second-Order Filter  Commented=through  FilterType=Low-pass  fn=initialFrequency  Zeta=1  Ts=sampleTime  A0=0  Ph0=0  f0=0  b0=0
  Switch : Switch  Criteria=u2 > Threshold  Threshold=1  SaturateOnIntegerOverflow=off  InputSameDT=off
  Freq : Outport
  wires:
  Second-Order Filter/1 -> Delay/1, Frequency estimation/1(sk), Hit Crossing/1
  Delay1/1 -> Frequency estimation/4(k-1)
  Hit Crossing/1 -> Frequency estimation/Trigger
  Delay/1 -> Frequency estimation/2(sk-1)
  V/1 -> Second-Order Filter/1
  Time/1 -> Switch/2, Delay1/1, Frequency estimation/3(k)
  Frequency estimation/1(f) -> Switch/1
  Constant1/1 -> Switch/3
  Switch/1 -> Freq/1

== system SimscapeCustomComponents_lib/Microgrid and Renewables/Storage/BESS Integrated/Detailed/BESS Controller/Grid Forming/Measurement/Frequency Measurement/Frequency Measurement/If Action Subsystem1 ==
  Action Port : ActionPort
  Constant1 : Constant  Value=initialFrequency
  Out1 : Outport
  wires:
  Constant1/1 -> Out1/1

== system SimscapeCustomComponents_lib/Microgrid and Renewables/Storage/BESS Integrated/Detailed/BESS Controller/Grid Forming/Measurement/Frequency Measurement/Frequency Measurement/Postive Sequence ==
  abc : Inport
  Complex to Real-Imag : ComplexToRealImag
  Demux : Demux  Outputs=3
  Symmetrical-Components Transform : eeTransforms/Symmetrical-Components Transform  PowerInvariant=off
  Terminator : Terminator
  Terminator1 : Terminator
  Terminator2 : Terminator
  Transpose : Math  Operator=transpose
  posSeq : Outport
  wires:
  Transpose/1 -> Symmetrical-Components Transform/1
  Symmetrical-Components Transform/1 -> Demux/1
  Complex to Real-Imag/1 -> posSeq/1
  Demux/1 -> Complex to Real-Imag/1
  abc/1 -> Transpose/1
  Complex to Real-Imag/2 -> Terminator/1
  Demux/2 -> Terminator1/1
  Demux/3 -> Terminator2/1

== system SimscapeCustomComponents_lib/Microgrid and Renewables/Storage/BESS Integrated/Detailed/BESS Controller/Grid Forming/Power Control/ActivePowerControl/vsmControl/Damping Frequency ==
  fref : Inport
  ConstantFreqReference : Subsystem  VariantControl=constFreq
  WithFrequencyMeasurement : Subsystem  VariantControl=freqMeas
  fmeas : Outport

== system SimscapeCustomComponents_lib/Microgrid and Renewables/Storage/BESS Integrated/Detailed/BESS Controller/Grid Forming/Power Control/ActivePowerControl/vsmControl/Power Reference Selection ==
  cntrlflag : Inport
  Pref : Inport  Port=2
  fref : Inport  Port=3
  Wsm : Inport  Port=4
  If : If
  If Action Subsystem : Subsystem  TreatAsAtomicUnit=on
  If Action Subsystem1 : Subsystem  TreatAsAtomicUnit=on
  Merge : Merge
  Scope : Scope
  power : Outport
  wires:
  If Action Subsystem1/1(Power) -> Merge/2
  If/1 -> If Action Subsystem/Action
  Pref/1 -> If Action Subsystem/1(Pref)
  [Wsm] -> If Action Subsystem1/2(Wsm)
  fref/1 -> If Action Subsystem1/1(fref)
  [Wsm] -> If Action Subsystem/2(Wsm)
  If Action Subsystem/1(Power) -> Merge/1
  If/2 -> If Action Subsystem1/Action
  cntrlflag/1 -> If/1
  Merge/1 -> Scope/1, power/1
  Wsm/1 -> [Wsm]

== system SimscapeCustomComponents_lib/Microgrid and Renewables/Storage/BESS Integrated/Detailed/BESS Controller/Grid Forming/Power Control/ReactiveControl/Voltage  Reference Selection/If Action Subsystem ==
  note: Vs-delV
  Qref : Inport
  Qmeas : Inport  Port=2
  Action Port : ActionPort
  Constant : Constant  Value=voltreference
  Gain : Gain  Gain=QVoltDroop
  Low-Pass Filter (Discrete or Continuous) : eeGeneralControl/Low-Pass Filter (Discrete or Continuous)  K=1  T=QVoltFilterTC  B=inf  A=-inf  init_option=Specify as parameter  x0=0  Ts=activePowerSampleTime
  Product1 : Product
  Scope : Scope
      settings: ActiveDisplayYMinimum=-0.00042  ActiveDisplayYMaximum=0.0007
  Scope1 : Scope  NumInputPorts=2
      settings: ActiveDisplayYMinimum=-0.71158  ActiveDisplayYMaximum=0.42604  DataLoggingVariableName=ScopeData5
  Sum : Sum  Inputs=|+-
  Sum1 : Sum  Inputs=|++
  Vd : Outport
  wires:
  Constant/1 -> Product1/2, Sum1/2
  Qmeas/1 -> Low-Pass Filter (Discrete or Continuous)/1, Scope1/2
  Gain/1 -> Scope/1, Sum1/1
  Qref/1 -> Sum/1, Scope1/1
  Low-Pass Filter (Discrete or Continuous)/1 -> Sum/2
  Sum/1 -> Gain/1
  Sum1/1 -> Product1/1
  Product1/1 -> Vd/1  "V"

== system SimscapeCustomComponents_lib/Microgrid and Renewables/Storage/BESS Integrated/Detailed/BESS Controller/Grid Forming/Power Control/ReactiveControl/Voltage  Reference Selection/If Action Subsystem1 ==
  note: Vs-delV
  Vref : Inport
  Vmeas : Inport  Port=2
  Action Port : ActionPort
  Constant : Constant  Value=voltreference
  Gain : Gain  Gain=1e-3/QVoltDroop
  Low-Pass Filter (Discrete or Continuous) : eeGeneralControl/Low-Pass Filter (Discrete or Continuous)  K=1  T=QVoltFilterTC  B=inf  A=-inf  init_option=Specify as parameter  x0=0  Ts=activePowerSampleTime
  Product1 : Product
  Scope : Scope
      settings: ActiveDisplayYMinimum=8.18716  ActiveDisplayYMaximum=11.15581  DataLoggingVariableName=ScopeData11  DataLoggingSaveFormat=Array
  Scope1 : Scope
      settings: ActiveDisplayYMinimum=0.78014  ActiveDisplayYMaximum=0.78049  DataLoggingVariableName=ScopeData12  DataLoggingSaveFormat=Array
  Scope2 : Scope  NumInputPorts=2
      settings: ActiveDisplayYMinimum=0.83186  ActiveDisplayYMaximum=1.08242  DataLoggingVariableName=ScopeData13  DataLoggingSaveFormat=Array
  Sum : Sum  Inputs=|+-
  Sum1 : Sum  Inputs=|++
  Voltage : Outport
  wires:
  Vref/1 -> Scope2/1, Product1/1, Sum/1
  Gain/1 -> Sum1/1
  Vmeas/1 -> Scope2/2, Low-Pass Filter (Discrete or Continuous)/1
  Constant/1 -> Sum1/2
  Low-Pass Filter (Discrete or Continuous)/1 -> Sum/2, Scope1/1
  Sum/1 -> Gain/1
  Product1/1 -> Voltage/1, Scope/1  "V"
  Sum1/1 -> Product1/2

== system SimscapeCustomComponents_lib/Microgrid and Renewables/Sources/Solar Plant Integrated/Detailed/PV Plant & Controller/Controller/MPPT/Solar PV Controller/DC voltage controller & current reference/If Action Subsystem/Subsystem ==
  V mag : Inport
  iq ub : Inport  Port=2
  Q ref : Inport  Port=3
  Constant : Constant  Value=1e-3
  Data Type Conversion Inherited : simulink/Signal Attributes/Data Type Conversion Inherited  ConvertRealWorld=Real World Value  DoSatur=off
  Divide2 : Product  Inputs=*/
  Gain3 : Gain  Gain=-1
  Saturation Dynamic2 : simulink/Discontinuities/Saturation Dynamic  OutMin=[]  OutMax=[]  OutDataTypeStr=Inherit: Same as second input  OutDataType=fixdt(1, 16)  OutScaling=2^-10  DoSatur=off
  Switch : Switch  Criteria=u2 ~= 0  SaturateOnIntegerOverflow=off  InputSameDT=off
  iq ub1 : InportShadow  Port=2
  iqref : Outport
  wires:
  iq ub1/1 -> Gain3/1
  Divide2/1 -> Saturation Dynamic2/2
  Q ref/1 -> Divide2/1
  Gain3/1 -> Saturation Dynamic2/3
  iq ub/1 -> Saturation Dynamic2/1
  Saturation Dynamic2/1 -> iqref/1
  V mag/1 -> Data Type Conversion Inherited/1, Switch/2, Switch/1
  Switch/1 -> Divide2/2
  Constant/1 -> Data Type Conversion Inherited/2
  Data Type Conversion Inherited/1 -> Switch/3

== system SimscapeCustomComponents_lib/Microgrid and Renewables/Sources/Solar Plant Integrated/Detailed/PV Plant & Controller/Controller/MPPT/Solar PV Controller/DC voltage controller & current reference/If Action Subsystem/Subsystem1 ==
  Vmag : Inport
  P pv : Inport  Port=2
  vdc : Inport  Port=3
  vdc ref : Inport  Port=4
  id ub : Inport  Port=5
  Constant : Constant  Value=1e-3
  Constant4 : Constant  Value=0
  Data Type Conversion Inherited : simulink/Signal Attributes/Data Type Conversion Inherited  ConvertRealWorld=Real World Value  DoSatur=off
  Divide : Product  Inputs=/*
  Gain4 : Gain  Gain=1/(mVAbase)
  Saturation Dynamic1 : simulink/Discontinuities/Saturation Dynamic  OutMin=[]  OutMax=[]  OutDataTypeStr=Inherit: Same as second input  OutDataType=fixdt(1, 16)  OutScaling=2^-10  DoSatur=off
  Scope : Scope  NumInputPorts=2
      settings: ActiveDisplayYMinimum=-55957.97767  ActiveDisplayYMaximum=503630.2665
  Sum : Sum  Inputs=|++
  Switch : Switch  Criteria=u2 ~= 0  SaturateOnIntegerOverflow=off  InputSameDT=off
  V_dc_Controller1 : Subsystem
  idref : Outport
  wires:
  Constant4/1 -> Saturation Dynamic1/3
  P pv/1 -> Gain4/1
  V_dc_Controller1/1(Out1) -> Sum/2
  Sum/1 -> Saturation Dynamic1/2
  vdc ref/1 -> V_dc_Controller1/2(vdc ref), Scope/2
  id ub/1 -> Saturation Dynamic1/1
  Gain4/1 -> Divide/2
  Divide/1 -> Sum/1
  Saturation Dynamic1/1 -> idref/1
  vdc/1 -> V_dc_Controller1/1(vdc), Scope/1
  Vmag/1 -> Data Type Conversion Inherited/1, Switch/2, Switch/1
  Switch/1 -> Divide/1
  Constant/1 -> Data Type Conversion Inherited/2
  Data Type Conversion Inherited/1 -> Switch/3

== system SimscapeCustomComponents_lib/Microgrid and Renewables/Sources/Solar Plant Integrated/Detailed/PV Plant & Controller/Controller/MPPT/Solar PV Controller/DC voltage controller & current reference/Subsystem1/V_dc_Controller1 ==
  vdc : Inport
  vdc ref : Inport  Port=2
  Gain : Gain  Gain=1/VdcBase
  PID Controller : slpidlib/PID Controller  Controller=PID  Form=Parallel  TimeDomain=Discrete-time  UseExternalTs=off  SampleTime=-1  IntegratorMethod=Forward Euler  FilterMethod=Forward Euler  ControllerParametersSource=internal  P=Kpv  I=Kiv  UseKiTs=off  D=Kdv  UseExternalDerivativeSource=off  N=100  UseFilter=on  TunerSelectOption=Transfer Function Based (PID Tuner App)  ZeroCross=off  InitialConditionSource=internal  InitialConditionForIntegrator=0  InitialConditionForFilter=0  DifferentiatorICPrevScaledInput=0  ExternalReset=none  TrackingMode=off  Kt=1  LimitOutput=off  SatLimitsSource=internal  UpperSaturationLimit=iMax  LowerSaturationLimit=0  LinearizeAsGain=on  AntiWindupMode=clamping  Kb=1  LimitIntegrator=off  UpperIntegratorSaturationLimit=inf  LowerIntegratorSaturationLimit=-inf  POutMin=[]  POutMax=[]  IOutMin=[]  IOutMax=[]  DOutMin=[]  DOutMax=[]  NOutMin=[]  NOutMax=[]  SumOutMin=[]  SumOutMax=[]  SaturationOutMin=[]  SaturationOutMax=[]  PParamMin=[]  PParamMax=[]  IParamMin=[]  IParamMax=[]  DParamMin=[]  DParamMax=[]  NParamMin=[]  NParamMax=[]  KbParamMin=[]  KbParamMax=[]  KtParamMin=[]  KtParamMax=[]  KbOutMin=[]  KbOutMax=[]  KtOutMin=[]  KtOutMax=[]  IntegratorOutMin=[]  IntegratorOutMax=[]  FilterOutMin=[]  FilterOutMax=[]  SumI1OutMin=[]  SumI1OutMax=[]  SumI2OutMin=[]  SumI2OutMax=[]  SumI3OutMin=[]  SumI3OutMax=[]  SumI4OutMin=[]  SumI4OutMax=[]  SumDOutMin=[]  SumDOutMax=[]  DifferentiatorOutMin=[]  DifferentiatorOutMax=[]  FilterDiffOutCoefMin=[]  FilterDiffOutCoefMax=[]  ReciprocalOutMin=[]  ReciprocalOutMax=[]  SumDenOutMin=[]  SumDenOutMax=[]  SumNumOutMin=[]  SumNumOutMax=[]  DivideOutMin=[]  DivideOutMax=[]  UdiffTsProdOutMin=[]  UdiffTsProdOutMax=[]  NTsProdOutMin=[]  NTsProdOutMax=[]  UintegralTsProdOutMin=[]  UintegralTsProdOutMax=[]  UngainTsProdOutMin=[]  UngainTsProdOutMax=[]  ClampingZeroOutDataTypeStr=Inherit: Inherit via back propagation  ClampingZeroOutMin=[]  ClampingZeroOutMax=[]  FilterDenConstantOutDataTypeStr=Inherit: Inherit via back propagation  FilterDenConstantOutMin=[]  FilterDenConstantOutMax=[]  PCopyOutDataTypeStr=Inherit: Inherit via back propagation  PCopyOutMin=[]  PCopyOutMax=[]  NCopyOutDataTypeStr=Inherit: Inherit via back propagation  NCopyOutMin=[]  NCopyOutMax=[]  IntegratorContinuousStateAttributes=''  IntegratorStateMustResolveToSignalObject=off  IntegratorRTWStateStorageClass=Auto  FilterContinuousStateAttributes=''  FilterStateMustResolveToSignalObject=off  FilterRTWStateStorageClass=Auto  ParallelPVariant=InternalParameters  IdealPVariant=Disabled  IVariant=InternalParameters  DVariant=InternalParameters  IntegratorVariant=Discrete  SatVariant=Disabled  AWVariant=Passthrough  PCopyVariant=Disabled  TRVariant=Disabled  FdbkBlocksVariant=Forward  IdealPFdbkVariant=Disabled  SatFdbkVariant=Disabled  DerivativeFilterVariant=ForwardEulerFilter  NVariant=InternalParameters  NCopyVariant=Disabled  FilterICVariant=InternalICsFilter  IntegratorICVariant=InternalICs  ExternalResetVariant=Disabled  TRSumVariant=Passthrough  SumFdbkVariant=Disabled  SumVariant=Sum_PID  TsampFilterVariant=InternalTs  TsampNgainVariant=Passthrough  TsampIntegralVariant=Disabled_SignalSpec  ExternalSaturationOutDataTypeStr=Inherit: Same as second input  DerivativeSourceVariant=ErrorSignal  PreIntVariant=InternalPreInt
  Sum : Sum  Inputs=|+-
  Out1 : Outport
  wires:
  vdc/1 -> Sum/1
  vdc ref/1 -> Sum/2
  PID Controller/1 -> Out1/1
  Gain/1 -> PID Controller/1
  Sum/1 -> Gain/1

== system SimscapeCustomComponents_lib/Microgrid and Renewables/Sources/Solar Plant Integrated/Detailed/PV Plant & Controller/Controller/Power Reference/Power Reference Controller/Power Reference Controller/Reference Current/Current limits ==
  Imax : Inport
  iqref : Inport  Port=2
  idref : Inport  Port=3
  Constant8 : Constant  Value=0
  Constant9 : Constant  Value=0
  Scope : Scope
      settings: ActiveDisplayYMinimum=-0.15  ActiveDisplayYMaximum=1.35  DataLoggingVariableName=ScopeData3
  Scope1 : Scope
      settings: ActiveDisplayYMinimum=-0.08298  ActiveDisplayYMaximum=0.74678  DataLoggingVariableName=ScopeData4
  Sqrt : Sqrt
  Sqrt1 : Sqrt
  Square{1..4} (4 alike) : Math  Operator=square
  Step2 : Step  Time=0.01  SampleTime=Ts
  Step3 : Step  Time=0.01  SampleTime=Ts
  Sum6 : Sum  Inputs=|+-
  Sum9 : Sum  Inputs=|+-
  Switch1 : Switch  Threshold=.01  SaturateOnIntegerOverflow=off  InputSameDT=off
  Switch2 : Switch  Threshold=.01  SaturateOnIntegerOverflow=off  InputSameDT=off
  iubq : Outport
  iubd : Outport  Port=2
  wires:
  Sum9/1 -> Switch2/1
  Step3/1 -> Switch2/2
  Step2/1 -> Switch1/2
  Switch2/1 -> Sqrt1/1
  Square1/1 -> Sum6/1
  Switch1/1 -> Sqrt/1
  iqref/1 -> Square2/1
  Square3/1 -> Sum9/1
  Sum6/1 -> Switch1/1
  Square2/1 -> Sum6/2
  Constant8/1 -> Switch1/3
  Square4/1 -> Sum9/2
  Constant9/1 -> Switch2/3
  Sqrt/1 -> Scope/1, iubd/1
  Imax/1 -> Square3/1, Square1/1
  Sqrt1/1 -> Scope1/1, iubq/1
  idref/1 -> Square4/1
